simulink model "circular_buffer"  (R2017b)
settings: Solver=FixedStepAuto  StartTime=0.0  StopTime=1  FixedStep=0.1  RelTol=1e-3
PreLoadFcn:
  | bufferlength = 10;
libraries: simulink x1
settings Model: Creator=Z634594  LastModifiedBy=Z634594

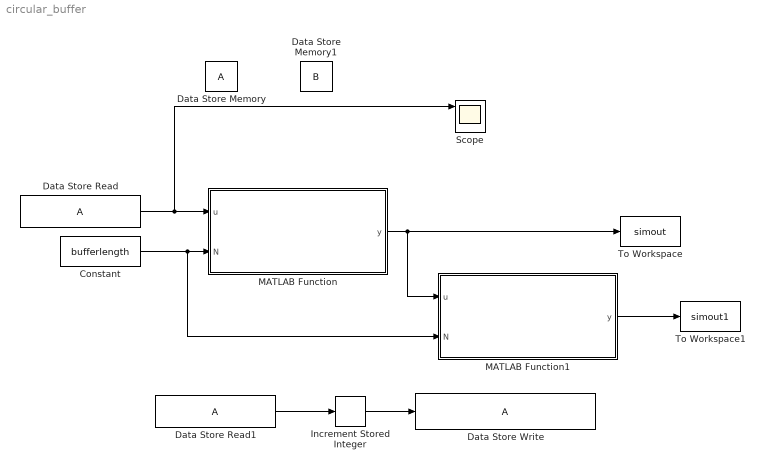
== system circular_buffer ==
  Constant : Constant  Value=bufferlength
  Data Store Memory : DataStoreMemory  ReadBeforeWriteMsg=warning  WriteAfterWriteMsg=warning  WriteAfterReadMsg=warning  InitialValue=[ 0 1 2 ]  ShowAdditionalParam=off
  Data Store Memory1 : DataStoreMemory  DataStoreName=B  ReadBeforeWriteMsg=warning  WriteAfterWriteMsg=warning  WriteAfterReadMsg=warning  InitialValue=[ 0 1 2 ]  ShowAdditionalParam=off
  Data Store Read : DataStoreRead  Priority=1
  Data Store Read1 : DataStoreRead  Priority=2
  Data Store Write : DataStoreWrite
  Increment Stored Integer : simulink/Additional Math & Discrete/Additional Math: Increment - Decrement/Increment Stored Integer
      settings: SourceProductName=Simulink
  MATLAB Function : MATLAB Function  TreatAsAtomicUnit=on
  MATLAB Function1 : MATLAB Function  TreatAsAtomicUnit=on
  Scope : Scope  NumInputPorts=3
  To Workspace : ToWorkspace  VariableName=simout  SaveFormat=Structure With Time  SampleTime=-1
  To Workspace1 : ToWorkspace  VariableName=simout1  SaveFormat=Structure With Time  SampleTime=-1
  wires:
  Data Store Read/1 -> Scope/1, MATLAB Function/1(u)
  Constant/1 -> MATLAB Function1/2(N), MATLAB Function/2(N)
  Increment Stored Integer/1 -> Data Store Write/1
  Data Store Read1/1 -> Increment Stored Integer/1
  MATLAB Function/1(y) -> MATLAB Function1/1(u), To Workspace/1
  MATLAB Function1/1(y) -> To Workspace1/1

== matlab function circular_buffer/MATLAB Function1 ==
  data: u input size=[bufferlength 3]; N input; y output size=[1 3]
function y = buffer_mean_value(u, N)
% Function to calculate the mean values of circular buffer columns

mean_value = [ sum(u(:,1))/N sum(u(:,2))/N sum(u(:,3))/N ];

% Output mean value
y = mean_value;

== matlab function circular_buffer/MATLAB Function ==
  data: u input; N input; y output size=[bufferlength 3]
function y = CircularBuffer(u, N)
% Function to implement a simple N element circular buffer
% Define the internal buffer variable as persistent so
% so that it will maintain its values from one time step
% to the next.

persistent buffer writeIdx

% Initialize the buffer the first time through
if isempty(buffer)
    % Initialize the buffer
    buffer = zeros(N,3);
    writeIdx = 1;
    buffer(writeIdx,:) = u;
    writeIdx = writeIdx+1;
else
    buffer(writeIdx,:) = u;
    if (writeIdx == N)
        writeIdx = 1;
    else
        writeIdx = writeIdx+1;
    end
end

% Output the buffer
y = buffer;
